simulink model "test6_2_v1_org"  (Simulink 10.0)
settings: Solver=ode45  StartTime=0.0  StopTime=50.0  RelTol=1e-3  EnableMultiTasking=on
libraries: dsparch4 x2, commrandsrc2 x1, commnoisgen2 x1
settings Model: Creator=asus  LastModifiedBy=bhisma
settings DataIOCC: LimitDataPoints=on
settings DebuggingCC: UnderspecifiedInitializationDetection=Simplified  MergeDetectMultiDrivingBlocksExec=error  SolverPrmCheckMsg=warning
settings GRTTargetCC: GeneratePreprocessorConditionals=Disable all  CombineOutputUpdateFcns=on  GRTInterface=off
settings ConfigComp: CovExternalEMLEnable=off  CovSFcnEnable=off

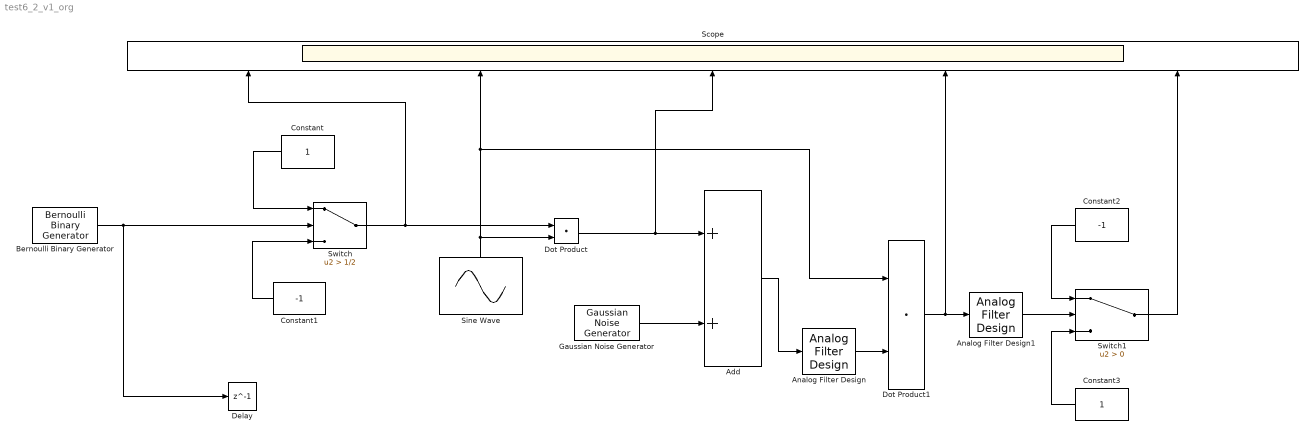
== system test6_2_v1_org ==
  Add : Sum
  Analog Filter Design : dsparch4/Analog Filter Design  method=Butterworth  filttype=Bandpass  N=8  Wlo=0.001  Whi=4*pi  Rp=2  Rs=40
  Analog Filter Design1 : dsparch4/Analog Filter Design  method=Butterworth  filttype=Lowpass  N=8  Wlo=4*pi  Whi=4*pi  Rp=2  Rs=40
  Bernoulli Binary Generator : commrandsrc2/Bernoulli Binary Generator  P=0.5  seed=61  Ts=1  frameBased=off  sampPerFrame=1  orient=off  outDataType=double
      settings: SourceProductName=Communications Toolbox  SourceProductBaseCode=CM
  Constant : Constant
  Constant1 : Constant  Value=-1
  Constant2 : Constant  Value=-1
  Constant3 : Constant
  Delay : Delay  DelayLength=1  InitialCondition=0
  Dot Product : DotProduct  InputSameDT=on  OutDataTypeStr=Inherit: Inherit via internal rule
  Dot Product1 : DotProduct  InputSameDT=on  OutDataTypeStr=Inherit: Inherit via internal rule
  Gaussian Noise Generator : commnoisgen2/Gaussian Noise Generator  m=0  d=1  s=41  Ts=1/50  frameBased=off  sampPerFrame=1  orient=off  outDataType=double
      settings: SourceProductName=Communications Toolbox  SourceProductBaseCode=CM
  Scope : Scope  NumInputPorts=5
  Sine Wave : Sin  Amplitude=5  Frequency=pi*2  SampleTime=1/8000
  Switch : Switch  Criteria=u2 > Threshold  Threshold=1/2
  Switch1 : Switch  Criteria=u2 > Threshold
  wires:
  Constant/1 -> Switch/1
  Constant1/1 -> Switch/3
  Bernoulli Binary Generator/1 -> Delay/1, Switch/2
  Switch/1 -> Scope/1, Dot Product/1
  Sine Wave/1 -> Scope/2, Dot Product1/1, Dot Product/2
  Gaussian Noise Generator/1 -> Add/2
  Dot Product/1 -> Scope/3, Add/1
  Dot Product1/1 -> Scope/4, Analog Filter Design1/1
  Analog Filter Design1/1 -> Switch1/2
  Constant2/1 -> Switch1/1
  Constant3/1 -> Switch1/3
  Switch1/1 -> Scope/5
  Add/1 -> Analog Filter Design/1
  Analog Filter Design/1 -> Dot Product1/2
